simulink model "MATE_IEEE123Node"  (R2024b)
settings: Solver=FixedStepDiscrete  StartTime=0.0  StopTime=1  FixedStep=Ts  RelTol=1e-3
PostLoadFcn:
  | Ts=50e-6;init_IEEE123Node;
InitFcn:
  | Ts=50e-6;init_IEEE123Node;
undefined symbols (not defined in the file): ft2km, loadcoeff, MATE, MATERT, Pa1, Pa13, Pa14, Pa17, Pa18, Pa22, Pa24, Pa25, Pa29, Pa31, Pa32, Pa33, Pa34, Pa35, Pa37, Pa38, Pa39, Pa44, Pa46, Pa48, Pa50, Pa51, Pa52, Pa53, Pa57, Pa59, Pa6, Pa61, Pa67, Pa7, Pa70, Pa73, Pa8, Pa81, Pa82, Pa83, Pa84, Pa85, Pa9, Pb10, Pb15, Pb2, Pb30, Pb33, Pb34, Pb35, Pb41, Pb42, Pb43, Pb47, Pb48, Pb57, Pb58, Pb60, Pb65, Pb66 ... (+124)
libraries: simetranss x259, ee_lib x93, fl_lib x67, nesl_utility x67, simetran x2
(part 3 of 4)

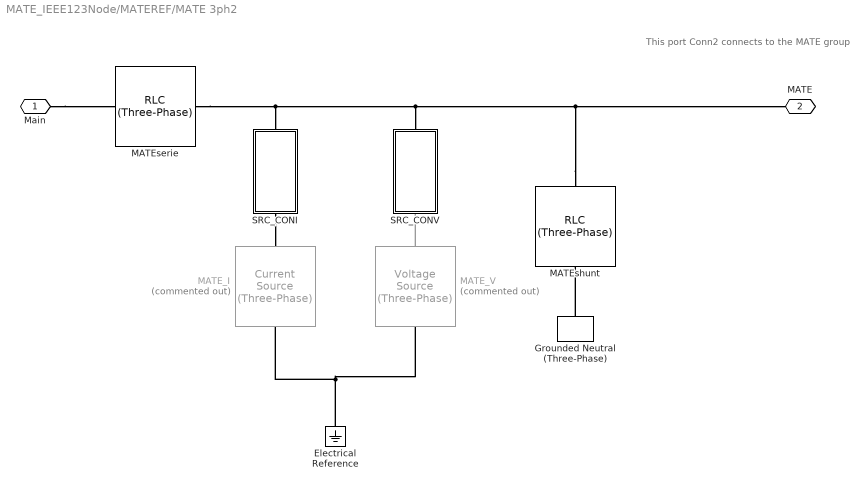
== system MATE_IEEE123Node/MATEREF/MATE 3ph2 ==
  note: This port Conn2 connects to the MATE group
  Electrical Reference : fl_lib/Electrical/Electrical Elements/Electrical Reference
  Grounded Neutral (Three-Phase) : ee_lib/Connectors & References/Grounded Neutral (Three-Phase)
  MATE_I : ee_lib/Sources/Current Source (Three-Phase)  Commented=on  iphase_rms=100 / sqrt(2) A  shift=0 deg  freq=60 Hz
      settings: InternalSimscapePortConfiguration="{\"Bottom\":[],\"Left\":[{\"id\":\"n\",\"label\":\"n\",\"type\":\"foundation.electrical.electrical\"}],\"Right\":[{\"id\":\"N\",\"label\":\"~\",\"type\":\"foundation.electrical.three_phase\"}],\"Top\":[]}"
  MATE_V : ee_lib/Sources/Voltage Source (Three-Phase)  Commented=on  vline_rms=0 V  shift=0 deg  freq=1 Hz  impedance_option=0  SShortCircuit=1e6 A*V  XR=15  R=0.0001 Ohm  L=3.97e-4 H  harmonic_option=0  harmonic_orders=[5, 7, 11, 13]  harmonic_ratios=[.1, .1, .1, .1]  G_parasitic=0 1/Ohm  I_specify=off  I_priority=None  I=[0, 0, 0] A  I_nominal_specify=off  I_nominal_value=1  I_nominal_unit=A
  MATEserie : ee_lib/Passive/RLC Assemblies/RLC (Three-Phase)  port_option=ee.enum.threePhasePort.composite  component_structure=ee.enum.rlc.structure.R  R=Rse Ohm  L=1e-3 H  C=1e-6 F  R_parasitic=0 Ohm  G_parasitic=0 1/Ohm  IL_specify=off  IL_priority=High  IL=[0, 0, 0] A  IL_nominal_specify=off  IL_nominal_value=1  IL_nominal_unit=A  VC_specify=off  VC_priority=High  VC=[0, 0, 0] V  VC_nominal_specify=off  VC_nominal_value=1  VC_nominal_unit=V
      settings: InternalSimscapePortConfiguration="{\"Bottom\":[],\"Left\":[{\"id\":\"N1\",\"label\":\"~1\",\"type\":\"foundation.electrical.three_phase\"}],\"Right\":[{\"id\":\"N2\",\"label\":\"~2\",\"type\":\"foundation.electrical.three_phase\"}],\"Top\":[]}"
  MATEshunt : ee_lib/Passive/RLC Assemblies/RLC (Three-Phase)  port_option=ee.enum.threePhasePort.composite  component_structure=ee.enum.rlc.structure.R  R=Rsh Ohm  L=1e-3 H  C=1e-6 F  R_parasitic=0 Ohm  G_parasitic=0 1/Ohm  IL_specify=off  IL_priority=High  IL=[0, 0, 0] A  IL_nominal_specify=off  IL_nominal_value=1  IL_nominal_unit=A  VC_specify=off  VC_priority=High  VC=[0, 0, 0] V  VC_nominal_specify=off  VC_nominal_value=1  VC_nominal_unit=V
      settings: InternalSimscapePortConfiguration="{\"Bottom\":[],\"Left\":[{\"id\":\"N1\",\"label\":\"~1\",\"type\":\"foundation.electrical.three_phase\"}],\"Right\":[{\"id\":\"N2\",\"label\":\"~2\",\"type\":\"foundation.electrical.three_phase\"}],\"Top\":[]}"
  SRC_CONI : Subsystem
  SRC_CONV : Subsystem
  Main : PMIOPort  Side=Left
  MATE : PMIOPort  Port=2  Side=Right
  connections:
  Main/RConn1 -- MATEserie/LConn1
  Grounded Neutral (Three-Phase)/LConn1 -- MATEshunt/LConn1
  SRC_CONI/RConn1 -- MATE_I/RConn1
  MATE_V/RConn1 -- SRC_CONV/RConn1
  MATE_V/LConn1 -- MATE_I/LConn1 -- Electrical Reference/LConn1
  MATEshunt/RConn1 -- MATE/RConn1 -- SRC_CONV/LConn1 -- MATEserie/RConn1 -- SRC_CONI/LConn1

== system MATE_IEEE123Node/MATEREF/sph ==
  Phase Splitter2 : ee_lib/Connectors & References/Phase Splitter
  abc : PMIOPort  Side=Left
  b : PMIOPort  Port=2  Side=Right
  connections:
  abc/RConn1 -- Phase Splitter2/LConn1
  b/RConn1 -- Phase Splitter2/RConn2

== system MATE_IEEE123Node/MATEREF/sph1 ==
  Phase Splitter2 : ee_lib/Connectors & References/Phase Splitter
  abc : PMIOPort  Side=Left
  b : PMIOPort  Port=2  Side=Right
  connections:
  b/RConn1 -- Phase Splitter2/RConn2
  abc/RConn1 -- Phase Splitter2/LConn1

== system MATE_IEEE123Node/MATEREF/sph2 ==
  Phase Splitter2 : ee_lib/Connectors & References/Phase Splitter
  abc : PMIOPort  Side=Left
  b : PMIOPort  Port=2  Side=Right
  connections:
  abc/RConn1 -- Phase Splitter2/LConn1
  b/RConn1 -- Phase Splitter2/RConn2

== system MATE_IEEE123Node/MATEREF/sph24 ==
  Phase Splitter2 : ee_lib/Connectors & References/Phase Splitter
  abc : PMIOPort  Side=Left
  c : PMIOPort  Port=2  Side=Right
  connections:
  abc/RConn1 -- Phase Splitter2/LConn1
  c/RConn1 -- Phase Splitter2/RConn3

== system MATE_IEEE123Node/MATEREF/sph25 ==
  Phase Splitter2 : ee_lib/Connectors & References/Phase Splitter
  abc : PMIOPort  Side=Left
  a : PMIOPort  Port=2  Side=Right
  connections:
  abc/RConn1 -- Phase Splitter2/LConn1
  a/RConn1 -- Phase Splitter2/RConn1

== system MATE_IEEE123Node/MATEREF/sph26 ==
  Phase Splitter2 : ee_lib/Connectors & References/Phase Splitter
  abc : PMIOPort  Side=Left
  b : PMIOPort  Port=2  Side=Right
  connections:
  abc/RConn1 -- Phase Splitter2/LConn1
  b/RConn1 -- Phase Splitter2/RConn2

== system MATE_IEEE123Node/MATEREF/sph27 ==
  Phase Splitter2 : ee_lib/Connectors & References/Phase Splitter
  abc : PMIOPort  Side=Left
  c : PMIOPort  Port=2  Side=Right
  connections:
  c/RConn1 -- Phase Splitter2/RConn3
  abc/RConn1 -- Phase Splitter2/LConn1

== system MATE_IEEE123Node/MATEREF/sph28 ==
  Phase Splitter2 : ee_lib/Connectors & References/Phase Splitter
  abc : PMIOPort  Side=Left
  b : PMIOPort  Port=2  Side=Right
  connections:
  b/RConn1 -- Phase Splitter2/RConn2
  abc/RConn1 -- Phase Splitter2/LConn1

== system MATE_IEEE123Node/MATEREF/sph29 ==
  Phase Splitter2 : ee_lib/Connectors & References/Phase Splitter
  abc : PMIOPort  Side=Left
  a : PMIOPort  Port=2  Side=Right
  connections:
  a/RConn1 -- Phase Splitter2/RConn1
  abc/RConn1 -- Phase Splitter2/LConn1

== system MATE_IEEE123Node/MATEREF/sph3 ==
  Phase Splitter2 : ee_lib/Connectors & References/Phase Splitter
  abc : PMIOPort  Side=Left
  b : PMIOPort  Port=2  Side=Right
  connections:
  abc/RConn1 -- Phase Splitter2/LConn1
  b/RConn1 -- Phase Splitter2/RConn2

== system MATE_IEEE123Node/MATEREF/sph30 ==
  Phase Splitter2 : ee_lib/Connectors & References/Phase Splitter
  abc : PMIOPort  Side=Left
  a : PMIOPort  Port=2  Side=Right
  connections:
  abc/RConn1 -- Phase Splitter2/LConn1
  a/RConn1 -- Phase Splitter2/RConn1

== system MATE_IEEE123Node/MATEREF/sph4 ==
  Phase Splitter2 : ee_lib/Connectors & References/Phase Splitter
  abc : PMIOPort  Side=Left
  b : PMIOPort  Port=2  Side=Right
  connections:
  b/RConn1 -- Phase Splitter2/RConn2
  abc/RConn1 -- Phase Splitter2/LConn1

== system MATE_IEEE123Node/MATEREF/sph42 ==
  Phase Splitter2 : ee_lib/Connectors & References/Phase Splitter
  abc : PMIOPort  Side=Left
  b : PMIOPort  Port=2  Side=Right
  connections:
  abc/RConn1 -- Phase Splitter2/LConn1
  b/RConn1 -- Phase Splitter2/RConn2

== system MATE_IEEE123Node/MATEREF/sph43 ==
  Phase Splitter2 : ee_lib/Connectors & References/Phase Splitter
  abc : PMIOPort  Side=Left
  a : PMIOPort  Port=2  Side=Right
  connections:
  a/RConn1 -- Phase Splitter2/RConn1
  abc/RConn1 -- Phase Splitter2/LConn1

== system MATE_IEEE123Node/MATEREF/sph44 ==
  Phase Splitter2 : ee_lib/Connectors & References/Phase Splitter
  abc : PMIOPort  Side=Left
  a : PMIOPort  Port=2  Side=Right
  connections:
  abc/RConn1 -- Phase Splitter2/LConn1
  a/RConn1 -- Phase Splitter2/RConn1

== system MATE_IEEE123Node/MATEREF/sph5 ==
  Phase Splitter2 : ee_lib/Connectors & References/Phase Splitter
  abc : PMIOPort  Side=Left
  c : PMIOPort  Port=2  Side=Right
  connections:
  abc/RConn1 -- Phase Splitter2/LConn1
  Phase Splitter2/RConn3 -- c/RConn1

== system MATE_IEEE123Node/MATEREF/sph51 ==
  Phase Splitter2 : ee_lib/Connectors & References/Phase Splitter
  abc : PMIOPort  Side=Left
  a : PMIOPort  Port=2  Side=Right
  connections:
  a/RConn1 -- Phase Splitter2/RConn1
  abc/RConn1 -- Phase Splitter2/LConn1

== system MATE_IEEE123Node/MATEREF/sph6 ==
  Phase Splitter2 : ee_lib/Connectors & References/Phase Splitter
  abc : PMIOPort  Side=Left
  a : PMIOPort  Port=2  Side=Right
  connections:
  abc/RConn1 -- Phase Splitter2/LConn1
  a/RConn1 -- Phase Splitter2/RConn1

== system MATE_IEEE123Node/MATEREF/sph7 ==
  Phase Splitter2 : ee_lib/Connectors & References/Phase Splitter
  abc : PMIOPort  Side=Left
  b : PMIOPort  Port=2  Side=Right
  connections:
  abc/RConn1 -- Phase Splitter2/LConn1
  b/RConn1 -- Phase Splitter2/RConn2

== system MATE_IEEE123Node/MATEREF/sph8 ==
  Phase Splitter2 : ee_lib/Connectors & References/Phase Splitter
  abc : PMIOPort  Side=Left
  a : PMIOPort  Port=2  Side=Right
  connections:
  a/RConn1 -- Phase Splitter2/RConn1
  abc/RConn1 -- Phase Splitter2/LConn1

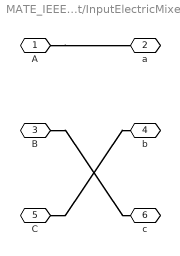
== system MATE_IEEE123Node/MATE_Equivalent/InputElectricMixer ==
  A : PMIOPort  Side=Left
  a : PMIOPort  Port=2  Side=Right
  B : PMIOPort  Port=3  Side=Left
  b : PMIOPort  Port=4  Side=Right
  C : PMIOPort  Port=5  Side=Left
  c : PMIOPort  Port=6  Side=Right
  connections:
  A/RConn1 -- a/RConn1
  B/RConn1 -- c/RConn1
  C/RConn1 -- b/RConn1

== system MATE_IEEE123Node/MATE_Equivalent/InternalSourceMixer ==
  0 : Constant  Value=-MATERT.SwitchVf./MATERT.Rsw  VectorParams1D=off
  1 : Constant  Value=ones(1,MATE.NumberOfNodes)  VectorParams1D=off
  Mux : Mux  Inputs=3
  Selector1 : Selector  Commented=on  InputPortWidth=size(MATE.source_parameter,1)+size(MATE.switch_parameter,1)  IndexOptions=Index vector (dialog)  Indices=MATE.src_Selector  OutputSizes=1
  sin : Sin  Amplitude=MATE.srcParam(1,:)  Frequency=MATE.srcParam(3,:)*2*pi  Phase=MATE.srcParam(2,:)*pi/180  SampleTime=Ts
  Out1 : Outport
  wires:
  sin/1 -> Mux/2
  0/1 -> Mux/1
  Mux/1 -> Out1/1
  1/1 -> Mux/3

== system MATE_IEEE123Node/MATE_Equivalent/InternalSwitchMixer ==
  Mux2 : Mux  Inputs=2
  Selector7 : Selector  InputPortWidth=1  IndexOptions=Index vector (dialog)  Indices="[ 1  1  1 ]"  OutputSizes=1
  gate : Outport
  wires:
  Selector7/1 -> Mux2/1
  [a58fxa8a9x743c756a9e3e] -> Selector7/1
  Mux2/1 -> gate/1
  [ae38xba66x2f62aef96d10] -> Mux2/2

== system MATE_IEEE123Node/MATE_Equivalent/MATEOutputSelector ==
  Yout : Inport
  BusCreator : BusCreator  Inputs=25
  Demux : Demux  Outputs=25
  SigOut : Outport
  wires:
  Demux/1 -> BusCreator/1  "SW_voltage:_1_CircuitBreaker3ph"
  Demux/2 -> BusCreator/2  "SW_voltage:_2_CircuitBreaker3ph"
  Demux/3 -> BusCreator/3  "SW_voltage:_3_CircuitBreaker3ph"
  Demux/4 -> BusCreator/4  "SW_voltage:_4_Switch"
  Demux/5 -> BusCreator/5  "Voltage:_5_CV_xfo"
  Demux/6 -> BusCreator/6  "Voltage:_6_CV_xfo"
  Demux/7 -> BusCreator/7  "Voltage:_7_CV_xfo"
  Demux/8 -> BusCreator/8  "Voltage:_8_bus13VI"
  Demux/9 -> BusCreator/9  "Voltage:_9_bus13VI"
  Demux/10 -> BusCreator/10  "Voltage:_10_bus13VI"
  Demux/11 -> BusCreator/11  "current:_11_CV_xfo"
  Demux/12 -> BusCreator/12  "current:_12_CV_xfo"
  Demux/13 -> BusCreator/13  "current:_13_CV_xfo"
  Demux/14 -> BusCreator/14  "current:_14_bus13VI"
  Demux/15 -> BusCreator/15  "current:_15_bus13VI"
  Demux/16 -> BusCreator/16  "current:_16_bus13VI"
  Demux/17 -> BusCreator/17  "MATEOut:_17_internal"
  Demux/18 -> BusCreator/18  "MATEOut:_18_internal"
  Demux/19 -> BusCreator/19  "MATEOut:_19_internal"
  Demux/20 -> BusCreator/20  "MATEOut:_20_internal"
  Demux/21 -> BusCreator/21  "MATEOut:_21_internal"
  Demux/22 -> BusCreator/22  "MATEOut:_22_internal"
  Demux/23 -> BusCreator/23  "MATEOut:_23_internal"
  Demux/24 -> BusCreator/24  "MATEOut:_24_internal"
  Demux/25 -> BusCreator/25  "MATEOut:_25_internal"
  BusCreator/1 -> SigOut/1
  Yout/1 -> Demux/1

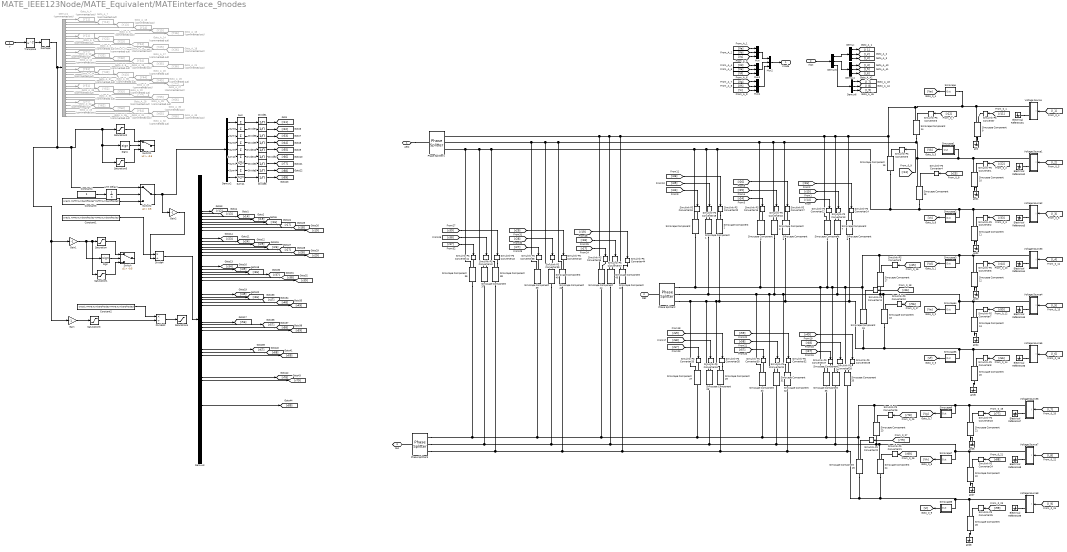
== system MATE_IEEE123Node/MATE_Equivalent/MATEinterface_9nodes ==
  Y : Inport
  Ihist : Inport  Port=2
  Constant1 : Constant  Value=ones(1,MATE.NumberOfNodes*MATE.NumberOfNodes)
  Constant2 : Constant  Value=ones(1,MATE.NumberOfNodes*MATE.NumberOfNodes)
  Constant3 : Constant  Value=ones(1,MATE.NumberOfNodes*MATE.NumberOfNodes)
  Constant4 : Constant
  Demux : Demux  Outputs=3
      settings: DisplayOption=none
  Demux1 : Demux  Commented=on  Outputs=36
      settings: DisplayOption=none
  Demux2 : Demux  Outputs="[9 9 9  9 9 9  9 9 9]"
      settings: DisplayOption=none
  Demux3 : Demux  Outputs=81
      settings: DisplayOption=none
  Demux4 : Demux  Outputs=3
      settings: DisplayOption=none
  Demux5 : Demux  Outputs=[3 3 3]
      settings: DisplayOption=none
  Demux6 : Demux  Outputs=3
      settings: DisplayOption=none
  Divide{1..3,5..11} (10 alike) : Product  Inputs=/
  Divide12 : Product  Inputs=*/  CollapseMode=Specified dimension
  Divide4 : Product  Inputs=*/  CollapseMode=Specified dimension
  Electrical Reference{1..9} (9 alike) : fl_lib/Electrical/Electrical Elements/Electrical Reference
  Gain : Gain  Gain=-1
  Gain1 : Gain  Gain=-1
  Gain2 : Gain  Gain=-1
  Goto_A_10 : Goto  Commented=on  GotoTag=Y23
  Goto_A_11 : Goto  Commented=on  GotoTag=Y31
  Goto_A_12 : Goto  Commented=on  GotoTag=Y32
  Goto_A_13 : Goto  Commented=on  GotoTag=Y14
  Goto_A_14 : Goto  Commented=on  GotoTag=Y15
  Goto_A_15 : Goto  Commented=on  GotoTag=Y16
  Goto_A_16 : Goto  Commented=on  GotoTag=Y24
  Goto_A_17 : Goto  Commented=on  GotoTag=Y25
  Goto_A_18 : Goto  Commented=on  GotoTag=Y26
  Goto_A_19 : Goto  Commented=on  GotoTag=Y34
  Goto_A_20 : Goto  Commented=on  GotoTag=Y35
  Goto_A_21 : Goto  Commented=on  GotoTag=Y36
  Goto_A_22 : Goto  Commented=on  GotoTag=Y53
  Goto_A_23 : Goto  Commented=on  GotoTag=Y61
  Goto_A_24 : Goto  Commented=on  GotoTag=Y62
  Goto_A_25 : Goto  Commented=on  GotoTag=Y44
  Goto_A_26 : Goto  Commented=on  GotoTag=Y45
  Goto_A_27 : Goto  Commented=on  GotoTag=Y46
  Goto_A_28 : Goto  Commented=on  GotoTag=Y54
  Goto_A_29 : Goto  Commented=on  GotoTag=Y55
  Goto_A_30 : Goto  Commented=on  GotoTag=Y66
  Goto_A_31 : Goto  Commented=on  GotoTag=Y64
  Goto_A_32 : Goto  Commented=on  GotoTag=Y65
  Goto_A_33 : Goto  Commented=on  GotoTag=Y66
  Goto_A_34 : Goto  Commented=on  GotoTag=Y41
  Goto_A_35 : Goto  Commented=on  GotoTag=Y52
  Goto_A_36 : Goto  Commented=on  GotoTag=Y63
  Goto_A_37 : Goto  Commented=on  GotoTag=Y42
  Goto_A_38 : Goto  Commented=on  GotoTag=Y43
  Goto_A_39 : Goto  Commented=on  GotoTag=Y51
  Goto_A_4 : Goto  Commented=on  GotoTag=Y11
  Goto_A_5 : Goto  Commented=on  GotoTag=Y22
  Goto_A_6 : Goto  Commented=on  GotoTag=Y33
  Goto_A_7 : Goto  Commented=on  GotoTag=Y12
  Goto_A_8 : Goto  Commented=on  GotoTag=Y13
  Goto_A_9 : Goto  Commented=on  GotoTag=Y21
  Mux : Mux  Inputs=3
  Mux1 : Mux  Inputs=3
  Mux2 : Mux  Inputs=[3 3 3]
  Mux4 : Mux  Inputs=3
  Phase Splitter1 : ee_lib/Connectors & References/Phase Splitter
  Phase Splitter2 : ee_lib/Connectors & References/Phase Splitter
  Phase Splitter3 : ee_lib/Connectors & References/Phase Splitter
  Reshape : Reshape
  Saturation : Saturate  UpperLimit=1e12  LowerLimit=1e-12
  Saturation1 : Saturate  UpperLimit=-1e-12  LowerLimit=-1e12
  Saturation2 : Saturate  UpperLimit=1e12  LowerLimit=1e-12
  Saturation3 : Saturate  UpperLimit=1e15  LowerLimit=-1e15
  Saturation4 : Saturate  UpperLimit=1e15  LowerLimit=-1e15
  Saturation5 : Saturate  UpperLimit=-1e-12  LowerLimit=-1e12
  Sign : Signum
  Sign1 : Signum
  Simscape : Subsystem
      mask Display: disp('V')
  Simscape Component{,1..44} (45 alike) : SimscapeComponentBlock  SourceFile=variable_resistor_unlimited  ComponentPath=variable_resistor_unlimited  ComponentVariants="[\"variable_resistor_unlimited\"]"  ComponentVariantNames="[\"variable_resistor_unlimited\"]"  ClassName=variable_resistor_unlimited  SchemaVersion=1  R0=0 Ohm  Rmaxp=1e9 Ohm  Rmaxn=-1e9 Ohm  Rminp=1e-9 Ohm  Rminn=-1e-9 Ohm  i_specify=off  i_priority=None  i=0 A  i_nominal_specify=off  i_nominal_value=1  i_nominal_unit=A  v_specify=off  v_priority=None  v=0 V  v_nominal_specify=off  v_nominal_value=1  v_nominal_unit=V
      settings: CopyFcn=simscape.engine.sli.internal.componentblockcallback(gcbh,'COPY')  PreCopyFcn=simscape.engine.sli.internal.componentblockcallback(gcbh,'PRECOPY')  PreDeleteFcn=simscape.engine.sli.internal.componentblockcallback(gcbh,'PREDELETE')  InternalSimscapePortConfiguration="{\"Bottom\":[],\"Left\":[{\"id\":\"R\",\"label\":\"R\",\"type\":\"input\"},{\"id\":\"p\",\"label\":\"+\",\"type\":\"foundation.electrical.electrical\"}],\"Right\":[{\"id\":\"n\",\"label\":\"-\",\"type\":\"foundation.electrical.electrical\"}],\"Top\":[]}"
      mask Type: Variable Resistor
  Simscape1 : Subsystem
      mask Display: disp('V')
  Simscape2 : Subsystem
      mask Display: disp('V')
  Simscape3 : Subsystem
      mask Display: disp('V')
  Simscape4 : Subsystem
      mask Display: disp('V')
  Simscape5 : Subsystem
      mask Display: disp('V')
  Simscape6 : Subsystem
      mask Display: disp('V')
  Simscape7 : Subsystem
      mask Display: disp('V')
  Simscape8 : Subsystem
      mask Display: disp('V')
  Simulink-PS Converter{,1..44} (45 alike) : nesl_utility/Simulink-PS Converter  PhysicalDomain=network_engine_domain  SubClassName=ps_input  LeftPortType=input  RightPortType=output  PseudoPeriodic=off  Frequencies=[]  NoiseDistribution=none  NoiseParameters=[]  Unit=1  AffineConversion=off  FilteringAndDerivatives=provide  SimscapeFilterOrder=1  InputFilterTimeConstant=0.001  UdotUserProvided=0
  Sum{,1..2,4..11} (11 alike) : Sum  Inputs=+
  Switch : Switch  Criteria=u2 > Threshold  Threshold=-0.5  SaturateOnIntegerOverflow=off  InputSameDT=off
  Switch1 : Switch  Criteria=u2 > Threshold  Threshold=-0.5  SaturateOnIntegerOverflow=off  InputSameDT=off
  Switch2 : Switch  Criteria=u2 > Threshold  Threshold=0.5  SaturateOnIntegerOverflow=off  InputSameDT=off
  Transpose : Math  Operator=transpose
  Unit Delay1 : UnitDelay  SampleTime=Ts  HasFrameUpgradeWarning=on
  Voltage Source : Subsystem
  Voltage Source1 : Subsystem
  Voltage Source2 : Subsystem
  Voltage Source3 : Subsystem
  Voltage Source4 : Subsystem
  Voltage Source5 : Subsystem
  Voltage Source6 : Subsystem
  Voltage Source7 : Subsystem
  Voltage Source8 : Subsystem
  gnd{,1..8} (9 alike) : fl_lib/Electrical/Electrical Elements/Electrical Reference
  ABC : PMIOPort  Side=Right
  DEF : PMIOPort  Port=2  Side=Right
  GHI : PMIOPort  Port=3  Side=Right
  Vnode : Outport  VectorParamsAs1DForOutWhenUnconnected=off
  wires:
  Demux/3 -> [I_3]
  [Vc] -> Mux/3
  Demux/2 -> [I_2]
  [Vb] -> Mux/2
  Demux/1 -> [I_1]
  [Va] -> Mux/1
  [I_2] -> Voltage Source1/1(I)
  Simscape2/1(Out) -> [Vc]
  [I_3] -> Voltage Source2/1(I)
  Simscape/1(Out) -> [Va]
  Simscape1/1(Out) -> [Vb]
  [I_1] -> Voltage Source/1(I)
  Y/1 -> Transpose/1
  Demux1/1 -> Goto_A_4/1
  Demux1/2 -> Goto_A_7/1
  Demux1/3 -> Goto_A_8/1
  Transpose/1 -> Reshape/1
  [r11] -> Simulink-PS Converter/1
  Sum/1 -> Divide1/1
  Divide1/1 -> [r11]
  [r22] -> Simulink-PS Converter1/1
  [r33] -> Simulink-PS Converter2/1
  [r12] -> Simulink-PS Converter3/1
  [r23] -> Simulink-PS Converter4/1
  [r13] -> Simulink-PS Converter5/1
  Demux1/4 -> Goto_A_13/1
  Demux1/5 -> Goto_A_14/1
  Demux1/6 -> Goto_A_15/1
  Demux1/7 -> Goto_A_9/1
  Demux1/8 -> Goto_A_5/1
  Demux1/9 -> Goto_A_10/1
  Demux1/10 -> Goto_A_16/1
  Demux1/11 -> Goto_A_17/1
  Demux1/12 -> Goto_A_18/1
  Demux1/13 -> Goto_A_11/1
  Demux1/14 -> Goto_A_12/1
  Demux1/15 -> Goto_A_6/1
  Demux1/16 -> Goto_A_19/1
  Demux1/17 -> Goto_A_20/1
  Demux1/18 -> Goto_A_21/1
  Demux1/36 -> Goto_A_33/1
  Demux1/35 -> Goto_A_32/1
  Demux1/34 -> Goto_A_31/1
  Demux1/33 -> Goto_A_36/1
  Demux1/32 -> Goto_A_24/1
  Demux1/31 -> Goto_A_23/1
  Demux1/30 -> Goto_A_30/1
  Demux1/29 -> Goto_A_29/1
  Demux1/28 -> Goto_A_28/1
  Demux1/27 -> Goto_A_22/1
  Demux1/26 -> Goto_A_35/1
  Demux1/25 -> Goto_A_39/1
  Demux1/24 -> Goto_A_27/1
  Demux1/23 -> Goto_A_26/1
  Demux1/22 -> Goto_A_25/1
  Demux1/21 -> Goto_A_38/1
  Demux1/20 -> Goto_A_37/1
  Demux1/19 -> Goto_A_34/1
  Demux2/1 -> Sum/1
  Divide7/1 -> [r22]
  Sum6/1 -> Divide7/1
  Demux2/2 -> Sum6/1
  Sum7/1 -> Divide8/1
  Divide8/1 -> [r33]
  Demux2/3 -> Sum7/1
  Demux2/4 -> Sum8/1
  Divide9/1 -> [r44]
  Sum8/1 -> Divide9/1
  Sum9/1 -> Divide10/1
  Divide10/1 -> [r55]
  Demux2/5 -> Sum9/1
  Divide11/1 -> [r66]
  Sum10/1 -> Divide11/1
  Demux2/6 -> Sum10/1
  [r44] -> Simulink-PS Converter6/1
  [I_4] -> Voltage Source3/1(I)
  Simscape3/1(Out) -> [Vd]
  Simscape4/1(Out) -> [Ve]
  [I_5] -> Voltage Source4/1(I)
  [r55] -> Simulink-PS Converter7/1
  [r66] -> Simulink-PS Converter8/1
  [I_6] -> Voltage Source5/1(I)
  Simscape5/1(Out) -> [Vf]
  [r45] -> Simulink-PS Converter9/1
  [r56] -> Simulink-PS Converter10/1
  [r46] -> Simulink-PS Converter11/1
  [Vd] -> Mux1/1
  [Ve] -> Mux1/2
  [Vf] -> Mux1/3
  Demux4/1 -> [I_4]
  Demux4/2 -> [I_5]
  Demux4/3 -> [I_6]
  [r14] -> Simulink-PS Converter12/1
  [r15] -> Simulink-PS Converter13/1
  [r16] -> Simulink-PS Converter14/1
  [r26] -> Simulink-PS Converter17/1
  [r25] -> Simulink-PS Converter16/1
  [r24] -> Simulink-PS Converter15/1
  Mux/1 -> Mux2/1
  Mux1/1 -> Mux2/2
  Mux2/1 -> Vnode/1
  Ihist/1 -> Demux5/1
  Demux5/1 -> Demux/1
  Demux5/2 -> Demux4/1
  Demux3/2 -> [r12]
  Demux3/3 -> [r13]
  Demux3/4 -> [r14]
  Demux3/5 -> [r15]
  Demux3/6 -> [r16]
  Gain1/1 -> Sign/1, Saturation1/1, Saturation/1
  Constant1/1 -> Divide4/1
  [r36] -> Simulink-PS Converter20/1
  [r35] -> Simulink-PS Converter19/1
  [r34] -> Simulink-PS Converter18/1
  Sign/1 -> Switch/2
  Saturation/1 -> Switch/1
  Saturation1/1 -> Switch/3
  Sum1/1 -> Divide3/1
  Divide3/1 -> [r77]
  Demux2/7 -> Sum1/1
  Divide5/1 -> [r88]
  Sum4/1 -> Divide5/1
  Demux2/8 -> Sum4/1
  Sum11/1 -> Divide6/1
  Divide6/1 -> [r99]
  Demux2/9 -> Sum11/1
  Demux3/7 -> [r17]
  Demux3/8 -> [r18]
  Demux3/9 -> [r19]
  Demux3/12 -> [r23]
  Demux3/13 -> [r24]
  Demux3/14 -> [r25]
  Demux3/15 -> [r26]
  Demux3/18 -> [r29]
  Demux3/17 -> [r28]
  Demux3/16 -> [r27]
  Demux3/22 -> [r34]
  Demux3/23 -> [r35]
  Demux3/24 -> [r36]
  Demux3/25 -> [r37]
  Demux3/26 -> [r38]
  Demux3/27 -> [r39]
  Demux3/32 -> [r45]
  Demux3/33 -> [r46]
  Demux3/36 -> [r49]
  Demux3/35 -> [r48]
  Demux3/34 -> [r47]
  Demux3/42 -> [r56]
  Demux3/44 -> [r58]
  Demux3/45 -> [r59]
  Demux3/43 -> [r57]
  Demux3/54 -> [r69]
  Demux3/53 -> [r68]
  Demux3/52 -> [r67]
  Demux3/63 -> [r79]
  Demux3/62 -> [r78]
  Demux3/72 -> [r89]
  Mux4/1 -> Mux2/3
  [Vi] -> Mux4/3
  [Vh] -> Mux4/2
  [Vg] -> Mux4/1
  Demux6/3 -> [I_9]
  Demux6/2 -> [I_8]
  Demux6/1 -> [I_7]
  Demux5/3 -> Demux6/1
  [r79] -> Simulink-PS Converter22/1
  [r89] -> Simulink-PS Converter21/1
  [r78] -> Simulink-PS Converter26/1
  Simscape8/1(Out) -> [Vi]
  [I_9] -> Voltage Source8/1(I)
  [r99] -> Simulink-PS Converter25/1
  [r88] -> Simulink-PS Converter24/1
  [I_8] -> Voltage Source7/1(I)
  Simscape7/1(Out) -> [Vh]
  Simscape6/1(Out) -> [Vg]
  [I_7] -> Voltage Source6/1(I)
  [r77] -> Simulink-PS Converter23/1
  [r67] -> Simulink-PS Converter33/1
  [r68] -> Simulink-PS Converter34/1
  [r69] -> Simulink-PS Converter35/1
  [r57] -> Simulink-PS Converter30/1
  [r58] -> Simulink-PS Converter31/1
  [r59] -> Simulink-PS Converter32/1
  [r49] -> Simulink-PS Converter29/1
  [r48] -> Simulink-PS Converter28/1
  [r47] -> Simulink-PS Converter27/1
  [r17] -> Simulink-PS Converter36/1
  [r18] -> Simulink-PS Converter37/1
  [r19] -> Simulink-PS Converter44/1
  [r29] -> Simulink-PS Converter40/1
  [r28] -> Simulink-PS Converter39/1
  [r27] -> Simulink-PS Converter38/1
  [r39] -> Simulink-PS Converter43/1
  [r38] -> Simulink-PS Converter42/1
  [r37] -> Simulink-PS Converter41/1
  Divide12/1 -> Saturation4/1
  Saturation3/1 -> Divide12/2
  Constant2/1 -> Divide12/1
  Gain/1 -> Saturation3/1
  Divide4/1 -> Demux3/1
  Saturation5/1 -> Switch1/3
  Saturation2/1 -> Switch1/1
  Sign1/1 -> Switch1/2
  Reshape/1 -> Gain1/1, Gain/1, Saturation5/1, Sign1/1, Saturation2/1, Switch2/1, Demux1/1
  Switch2/1 -> Gain2/1, Demux2/1
  Unit Delay1/1 -> Switch2/2
  Constant4/1 -> Unit Delay1/1
  Constant3/1 -> Switch2/3
  Gain2/1 -> Divide4/2
  connections:
  Simscape Component14/LConn2 -- Simscape Component9/LConn2 -- Voltage Source/RConn1 -- Simscape/LConn1 -- Simscape Component16/LConn2 -- Simscape Component6/LConn2 -- Simscape Component7/LConn2 -- Simscape Component8/LConn2 -- Simscape Component42/LConn2 -- Simscape Component43/LConn2 -- Simscape Component44/LConn2 -- Phase Splitter1/RConn1
  Simscape Component11/LConn2 -- Voltage Source2/RConn1 -- Simscape2/LConn1 -- Simscape Component15/RConn1 -- Simscape Component16/RConn1 -- Simscape Component2/LConn2 -- Simscape Component1/LConn2 -- Simscape Component/LConn2 -- Simscape Component38/LConn2 -- Simscape Component37/LConn2 -- Simscape Component36/LConn2 -- Phase Splitter1/RConn3
  Simscape Component10/LConn2 -- Voltage Source1/RConn1 -- Simscape1/LConn1 -- Simscape Component15/LConn2 -- Simscape Component14/RConn1 -- Simscape Component5/LConn2 -- Simscape Component4/LConn2 -- Simscape Component3/LConn2 -- Simscape Component41/LConn2 -- Simscape Component40/LConn2 -- Simscape Component39/LConn2 -- Phase Splitter1/RConn2
  Electrical Reference2/LConn1 -- Voltage Source1/RConn2
  Electrical Reference3/LConn1 -- Voltage Source2/RConn2
  Electrical Reference1/LConn1 -- Voltage Source/RConn2
  ABC/RConn1 -- Phase Splitter1/LConn1
  Simscape Component9/RConn1 -- gnd/LConn1
  Simscape Component9/LConn1 -- Simulink-PS Converter/RConn1
  Simscape Component10/RConn1 -- gnd1/LConn1
  Simscape Component10/LConn1 -- Simulink-PS Converter1/RConn1
  Simscape Component11/RConn1 -- gnd2/LConn1
  Simscape Component11/LConn1 -- Simulink-PS Converter2/RConn1
  Simscape Component14/LConn1 -- Simulink-PS Converter3/RConn1
  Simscape Component15/LConn1 -- Simulink-PS Converter4/RConn1
  Simscape Component16/LConn1 -- Simulink-PS Converter5/RConn1
  Simscape Component17/LConn2 -- Simscape Component3/RConn1 -- Simscape Component/RConn1 -- Phase Splitter2/RConn1 -- Simscape Component35/LConn2 -- Simscape Component8/RConn1 -- Simscape Component34/LConn2 -- Simscape Component33/LConn2 -- Simscape Component19/LConn2 -- Simscape Component12/LConn2 -- Voltage Source3/RConn1 -- Simscape3/LConn1
  Simscape Component12/LConn1 -- Simulink-PS Converter6/RConn1
  Simscape Component12/RConn1 -- gnd3/LConn1
  Electrical Reference4/LConn1 -- Voltage Source3/RConn2
  Simscape Component13/LConn2 -- Voltage Source4/RConn1 -- Simscape4/LConn1 -- Simscape Component17/RConn1 -- Simscape Component1/RConn1 -- Phase Splitter2/RConn2 -- Simscape Component30/LConn2 -- Simscape Component31/LConn2 -- Simscape Component4/RConn1 -- Simscape Component32/LConn2 -- Simscape Component7/RConn1 -- Simscape Component18/LConn2
  Simscape Component13/RConn1 -- gnd4/LConn1
  Simscape Component13/LConn1 -- Simulink-PS Converter7/RConn1
  Electrical Reference5/LConn1 -- Voltage Source4/RConn2
  Simscape Component6/RConn1 -- Phase Splitter2/RConn3 -- Simscape Component27/LConn2 -- Simscape Component28/LConn2 -- Simscape Component29/LConn2 -- Simscape Component2/RConn1 -- Simscape Component5/RConn1 -- Simscape Component19/RConn1 -- Simscape Component18/RConn1 -- Simscape5/LConn1 -- Voltage Source5/RConn1 -- Simscape Component20/LConn2
  Electrical Reference6/LConn1 -- Voltage Source5/RConn2
  Simscape Component20/LConn1 -- Simulink-PS Converter8/RConn1
  Simscape Component20/RConn1 -- gnd5/LConn1
  Phase Splitter2/LConn1 -- DEF/RConn1
  Simscape Component17/LConn1 -- Simulink-PS Converter9/RConn1
  Simscape Component18/LConn1 -- Simulink-PS Converter10/RConn1
  Simscape Component19/LConn1 -- Simulink-PS Converter11/RConn1
  Simscape Component8/LConn1 -- Simulink-PS Converter12/RConn1
  Simscape Component7/LConn1 -- Simulink-PS Converter13/RConn1
  Simscape Component6/LConn1 -- Simulink-PS Converter14/RConn1
  Simscape Component3/LConn1 -- Simulink-PS Converter15/RConn1
  Simscape Component4/LConn1 -- Simulink-PS Converter16/RConn1
  Simscape Component5/LConn1 -- Simulink-PS Converter17/RConn1
  Simscape Component/LConn1 -- Simulink-PS Converter18/RConn1
  Simscape Component1/LConn1 -- Simulink-PS Converter19/RConn1
  Simulink-PS Converter20/RConn1 -- Simscape Component2/LConn1
  Simscape Component23/LConn2 -- Simscape Component36/RConn1 -- Phase Splitter3/RConn1 -- Simscape Component39/RConn1 -- Simscape Component44/RConn1 -- Simscape Component27/RConn1 -- Simscape Component30/RConn1 -- Simscape Component35/RConn1 -- Simscape Component25/LConn2 -- Simscape6/LConn1 -- Voltage Source6/RConn1 -- Simscape Component21/LConn2
  Simscape Component22/LConn2 -- Simscape Component24/LConn2 -- Simscape Component37/RConn1 -- Phase Splitter3/RConn2 -- Simscape Component40/RConn1 -- Simscape Component43/RConn1 -- Simscape Component28/RConn1 -- Simscape Component31/RConn1 -- Simscape Component34/RConn1 -- Simscape Component23/RConn1 -- Simscape7/LConn1 -- Voltage Source7/RConn1
  Simscape Component25/RConn1 -- Phase Splitter3/RConn3 -- Simscape Component38/RConn1 -- Simscape Component41/RConn1 -- Simscape Component42/RConn1 -- Simscape Component29/RConn1 -- Simscape Component32/RConn1 -- Simscape Component33/RConn1 -- Simscape Component26/LConn2 -- Voltage Source8/RConn1 -- Simscape8/LConn1 -- Simscape Component24/RConn1
  Simscape Component25/LConn1 -- Simulink-PS Converter22/RConn1
  Simscape Component23/LConn1 -- Simulink-PS Converter26/RConn1
  Simscape Component26/RConn1 -- gnd8/LConn1
  Electrical Reference9/LConn1 -- Voltage Source8/RConn2
  Simscape Component22/RConn1 -- gnd7/LConn1
  Electrical Reference7/LConn1 -- Voltage Source6/RConn2
  Electrical Reference8/LConn1 -- Voltage Source7/RConn2
  Simscape Component21/RConn1 -- gnd6/LConn1
  Simscape Component26/LConn1 -- Simulink-PS Converter25/RConn1
  Simscape Component24/LConn1 -- Simulink-PS Converter21/RConn1
  Simscape Component21/LConn1 -- Simulink-PS Converter23/RConn1
  Simscape Component22/LConn1 -- Simulink-PS Converter24/RConn1
  Phase Splitter3/LConn1 -- GHI/RConn1
  Simscape Component28/LConn1 -- Simulink-PS Converter34/RConn1
  Simscape Component27/LConn1 -- Simulink-PS Converter33/RConn1
  Simscape Component32/LConn1 -- Simulink-PS Converter32/RConn1
  Simscape Component31/LConn1 -- Simulink-PS Converter31/RConn1
  Simscape Component30/LConn1 -- Simulink-PS Converter30/RConn1
  Simscape Component33/LConn1 -- Simulink-PS Converter29/RConn1
  Simscape Component34/LConn1 -- Simulink-PS Converter28/RConn1
  Simscape Component35/LConn1 -- Simulink-PS Converter27/RConn1
  Simulink-PS Converter35/RConn1 -- Simscape Component29/LConn1
  Simulink-PS Converter43/RConn1 -- Simscape Component38/LConn1
  Simscape Component44/LConn1 -- Simulink-PS Converter36/RConn1
  Simulink-PS Converter44/RConn1 -- Simscape Component42/LConn1
  Simscape Component39/LConn1 -- Simulink-PS Converter38/RConn1
  Simscape Component40/LConn1 -- Simulink-PS Converter39/RConn1
  Simscape Component41/LConn1 -- Simulink-PS Converter40/RConn1
  Simscape Component36/LConn1 -- Simulink-PS Converter41/RConn1
  Simscape Component43/LConn1 -- Simulink-PS Converter37/RConn1
  Simscape Component37/LConn1 -- Simulink-PS Converter42/RConn1

== system MATE_IEEE123Node/NorthEast/28 ==
  Connection Port : PMIOPort  Side=Left
  Connection Port1 : PMIOPort  Port=2  Side=Right
  Connection Port2 : PMIOPort  Port=3  Side=Left
  Connection Port3 : PMIOPort  Port=4  Side=Right
  connections:
  Connection Port/RConn1 -- Connection Port1/RConn1
  Connection Port2/RConn1 -- Connection Port3/RConn1

== system MATE_IEEE123Node/NorthEast/sph21 ==
  Phase Splitter2 : ee_lib/Connectors & References/Phase Splitter
  abc : PMIOPort  Side=Left
  a : PMIOPort  Port=2  Side=Right
  connections:
  Phase Splitter2/RConn1 -- a/RConn1
  abc/RConn1 -- Phase Splitter2/LConn1

== system MATE_IEEE123Node/NorthEast/sph22 ==
  Phase Splitter2 : ee_lib/Connectors & References/Phase Splitter
  abc : PMIOPort  Side=Left
  a : PMIOPort  Port=2  Side=Right
  connections:
  abc/RConn1 -- Phase Splitter2/LConn1
  a/RConn1 -- Phase Splitter2/RConn1

== system MATE_IEEE123Node/NorthEast/sph23 ==
  Phase Splitter2 : ee_lib/Connectors & References/Phase Splitter
  abc : PMIOPort  Side=Left
  c : PMIOPort  Port=2  Side=Right
  connections:
  abc/RConn1 -- Phase Splitter2/LConn1
  Phase Splitter2/RConn3 -- c/RConn1

== system MATE_IEEE123Node/NorthEast/sph31 ==
  Phase Splitter2 : ee_lib/Connectors & References/Phase Splitter
  abc : PMIOPort  Side=Left
  a : PMIOPort  Port=2  Side=Right
  connections:
  abc/RConn1 -- Phase Splitter2/LConn1
  a/RConn1 -- Phase Splitter2/RConn1

== system MATE_IEEE123Node/NorthEast/sph32 ==
  Phase Splitter2 : ee_lib/Connectors & References/Phase Splitter
  abc : PMIOPort  Side=Left
  b : PMIOPort  Port=2  Side=Right
  connections:
  abc/RConn1 -- Phase Splitter2/LConn1
  Phase Splitter2/RConn2 -- b/RConn1

== system MATE_IEEE123Node/NorthEast/sph33 ==
  Phase Splitter2 : ee_lib/Connectors & References/Phase Splitter
  abc : PMIOPort  Side=Left
  c : PMIOPort  Port=2  Side=Right
  connections:
  abc/RConn1 -- Phase Splitter2/LConn1
  Phase Splitter2/RConn3 -- c/RConn1

== system MATE_IEEE123Node/NorthEast/sph34 ==
  Phase Splitter2 : ee_lib/Connectors & References/Phase Splitter
  abc : PMIOPort  Side=Left
  a : PMIOPort  Port=2  Side=Right
  c : PMIOPort  Port=3  Side=Right
  connections:
  Phase Splitter2/RConn3 -- c/RConn1
  abc/RConn1 -- Phase Splitter2/LConn1
  a/RConn1 -- Phase Splitter2/RConn1

== system MATE_IEEE123Node/NorthEast/sph35 ==
  Phase Splitter2 : ee_lib/Connectors & References/Phase Splitter
  abc : PMIOPort  Side=Left
  a : PMIOPort  Port=2  Side=Right
  connections:
  a/RConn1 -- Phase Splitter2/RConn1
  abc/RConn1 -- Phase Splitter2/LConn1

== system MATE_IEEE123Node/NorthEast/sph36 ==
  Phase Splitter2 : ee_lib/Connectors & References/Phase Splitter
  abc : PMIOPort  Side=Left
  a : PMIOPort  Port=2  Side=Right
  connections:
  abc/RConn1 -- Phase Splitter2/LConn1
  a/RConn1 -- Phase Splitter2/RConn1

== system MATE_IEEE123Node/NorthEast/sph37 ==
  Phase Splitter2 : ee_lib/Connectors & References/Phase Splitter
  abc : PMIOPort  Side=Left
  c : PMIOPort  Port=2  Side=Right
  connections:
  abc/RConn1 -- Phase Splitter2/LConn1
  Phase Splitter2/RConn3 -- c/RConn1

== system MATE_IEEE123Node/NorthEast/sph38 ==
  Phase Splitter2 : ee_lib/Connectors & References/Phase Splitter
  abc : PMIOPort  Side=Left
  c : PMIOPort  Port=2  Side=Right
  connections:
  abc/RConn1 -- Phase Splitter2/LConn1
  c/RConn1 -- Phase Splitter2/RConn3

== system MATE_IEEE123Node/NorthEast/sph39 ==
  Phase Splitter2 : ee_lib/Connectors & References/Phase Splitter
  abc : PMIOPort  Side=Left
  a : PMIOPort  Port=2  Side=Right
  b : PMIOPort  Port=3  Side=Right
  connections:
  b/RConn1 -- Phase Splitter2/RConn2
  abc/RConn1 -- Phase Splitter2/LConn1
  a/RConn1 -- Phase Splitter2/RConn1

== system MATE_IEEE123Node/NorthEast/sph40 ==
  Phase Splitter2 : ee_lib/Connectors & References/Phase Splitter
  abc : PMIOPort  Side=Left
  a : PMIOPort  Port=2  Side=Right
  connections:
  a/RConn1 -- Phase Splitter2/RConn1
  abc/RConn1 -- Phase Splitter2/LConn1

== system MATE_IEEE123Node/NorthEast/sph41 ==
  Phase Splitter2 : ee_lib/Connectors & References/Phase Splitter
  abc : PMIOPort  Side=Left
  a : PMIOPort  Port=2  Side=Right
  b : PMIOPort  Port=3  Side=Right
  connections:
  a/RConn1 -- Phase Splitter2/RConn1
  abc/RConn1 -- Phase Splitter2/LConn1
  Phase Splitter2/RConn2 -- b/RConn1

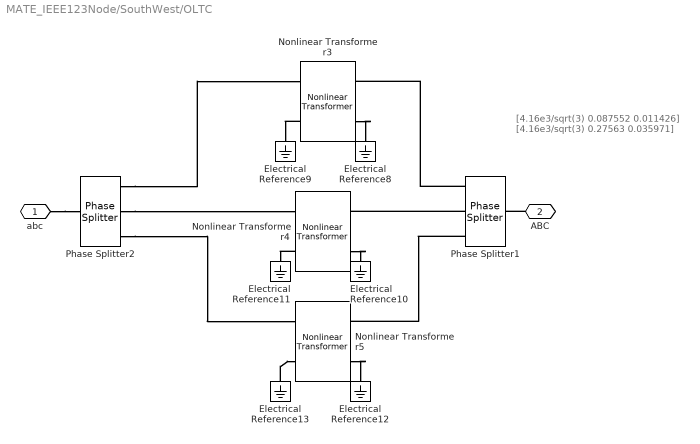
== system MATE_IEEE123Node/SouthWest/OLTC ==
  note: [4.16e3/sqrt(3) 0.087552 0.011426]
      | [4.16e3/sqrt(3) 0.27563 0.035971]
  Electrical Reference{8..13} (6 alike) : fl_lib/Electrical/Electrical Elements/Electrical Reference
  Nonlinear Transformer3 : ee_lib/Passive/Transformers/Nonlinear Transformer  Nw=1  Nw2=1  winding_param_option=2  Req=0.01 Ohm  Leq=0.0001 H  R_1=0.087552 Ohm  L_1=0.011426 H  R_2=0.27563 Ohm  L_2=0.035971 H  averaging_period=0 s  R_m=50000 Ohm  parameterization_option=1  H_data=[0, 200, 400, 600, 800, 1000] A/m  B_data=[0, .81, 1.25, 1.42, 1.48, 1.49] T  length_effective=0.2 m  area_effective=2e-4 m^2  L=1 H  L_sat=1e-2 H  current_data=[0, .4, .8, 1.2, 1.6, 2] A  magnetic_flux_data=[0, .161, .25, .284, .295, .299] .* 1e-3 Wb  magnetic_flux_sat=1.6e-04 Wb  dBdH0=0.005 T*m/A  B1=1.49 T  H1=1000 A/m  c=0.1  K=200 A/m  alpha=1e-4  interpolation_option=1  Leq_i0=0 A  L1_i0=0 A  L2_i0=0 A  x0_option=1  i_L0=0 A  phi0=0 Wb  B0=0 T  H0=0 A/m  Leq_g=1e-9 1/Ohm  L1_g=1e-9 1/Ohm  L2_g=1e-9 1/Ohm
      settings: InternalSimscapePortConfiguration="{\"Bottom\":[],\"Left\":[{\"id\":\"p1\",\"label\":\"1+\",\"type\":\"foundation.electrical.electrical\"},{\"id\":\"n1\",\"label\":\"1-\",\"type\":\"foundation.electrical.electrical\"}],\"Right\":[{\"id\":\"p2\",\"label\":\"2+\",\"type\":\"foundation.electrical.electrical\"},{\"id\":\"n2\",\"label\":\"2-\",\"type\":\"foundation.electrical.electrical\"}],\"Top\":[]}"
  Nonlinear Transformer4 : ee_lib/Passive/Transformers/Nonlinear Transformer  Nw=1  Nw2=1  winding_param_option=2  Req=0.01 Ohm  Leq=0.0001 H  R_1=0.087552 Ohm  L_1=0.011426 H  R_2=0.27563 Ohm  L_2=0.035971 H  averaging_period=0 s  R_m=50000 Ohm  parameterization_option=1  H_data=[0, 200, 400, 600, 800, 1000] A/m  B_data=[0, .81, 1.25, 1.42, 1.48, 1.49] T  length_effective=0.2 m  area_effective=2e-4 m^2  L=1 H  L_sat=1e-2 H  current_data=[0, .4, .8, 1.2, 1.6, 2] A  magnetic_flux_data=[0, .161, .25, .284, .295, .299] .* 1e-3 Wb  magnetic_flux_sat=1.6e-04 Wb  dBdH0=0.005 T*m/A  B1=1.49 T  H1=1000 A/m  c=0.1  K=200 A/m  alpha=1e-4  interpolation_option=1  Leq_i0=0 A  L1_i0=0 A  L2_i0=0 A  x0_option=1  i_L0=0 A  phi0=0 Wb  B0=0 T  H0=0 A/m  Leq_g=1e-9 1/Ohm  L1_g=1e-9 1/Ohm  L2_g=1e-9 1/Ohm
      settings: InternalSimscapePortConfiguration="{\"Bottom\":[],\"Left\":[{\"id\":\"p1\",\"label\":\"1+\",\"type\":\"foundation.electrical.electrical\"},{\"id\":\"n1\",\"label\":\"1-\",\"type\":\"foundation.electrical.electrical\"}],\"Right\":[{\"id\":\"p2\",\"label\":\"2+\",\"type\":\"foundation.electrical.electrical\"},{\"id\":\"n2\",\"label\":\"2-\",\"type\":\"foundation.electrical.electrical\"}],\"Top\":[]}"
  Nonlinear Transformer5 : ee_lib/Passive/Transformers/Nonlinear Transformer  Nw=1  Nw2=1  winding_param_option=2  Req=0.01 Ohm  Leq=0.0001 H  R_1=0.087552 Ohm  L_1=0.011426 H  R_2=0.27563 Ohm  L_2=0.035971 H  averaging_period=0 s  R_m=50000 Ohm  parameterization_option=1  H_data=[0, 200, 400, 600, 800, 1000] A/m  B_data=[0, .81, 1.25, 1.42, 1.48, 1.49] T  length_effective=0.2 m  area_effective=2e-4 m^2  L=1 H  L_sat=1e-2 H  current_data=[0, .4, .8, 1.2, 1.6, 2] A  magnetic_flux_data=[0, .161, .25, .284, .295, .299] .* 1e-3 Wb  magnetic_flux_sat=1.6e-04 Wb  dBdH0=0.005 T*m/A  B1=1.49 T  H1=1000 A/m  c=0.1  K=200 A/m  alpha=1e-4  interpolation_option=1  Leq_i0=0 A  L1_i0=0 A  L2_i0=0 A  x0_option=1  i_L0=0 A  phi0=0 Wb  B0=0 T  H0=0 A/m  Leq_g=1e-9 1/Ohm  L1_g=1e-9 1/Ohm  L2_g=1e-9 1/Ohm
      settings: InternalSimscapePortConfiguration="{\"Bottom\":[],\"Left\":[{\"id\":\"p1\",\"label\":\"1+\",\"type\":\"foundation.electrical.electrical\"},{\"id\":\"n1\",\"label\":\"1-\",\"type\":\"foundation.electrical.electrical\"}],\"Right\":[{\"id\":\"p2\",\"label\":\"2+\",\"type\":\"foundation.electrical.electrical\"},{\"id\":\"n2\",\"label\":\"2-\",\"type\":\"foundation.electrical.electrical\"}],\"Top\":[]}"
  Phase Splitter1 : ee_lib/Connectors & References/Phase Splitter
  Phase Splitter2 : ee_lib/Connectors & References/Phase Splitter
  abc : PMIOPort  Side=Left
  ABC : PMIOPort  Port=2  Side=Right
  connections:
  Nonlinear Transformer4/RConn2 -- Electrical Reference10/LConn1
  Nonlinear Transformer5/RConn2 -- Electrical Reference12/LConn1
  Electrical Reference13/LConn1 -- Nonlinear Transformer5/LConn2
  Nonlinear Transformer3/LConn2 -- Electrical Reference9/LConn1
  Nonlinear Transformer4/LConn2 -- Electrical Reference11/LConn1
  Nonlinear Transformer3/RConn2 -- Electrical Reference8/LConn1
  Phase Splitter2/RConn3 -- Nonlinear Transformer5/LConn1
  Phase Splitter2/RConn2 -- Nonlinear Transformer4/LConn1
  abc/RConn1 -- Phase Splitter2/LConn1
  Phase Splitter2/RConn1 -- Nonlinear Transformer3/LConn1
  ABC/RConn1 -- Phase Splitter1/LConn1
  Phase Splitter1/RConn1 -- Nonlinear Transformer3/RConn1
  Phase Splitter1/RConn2 -- Nonlinear Transformer4/RConn1
  Phase Splitter1/RConn3 -- Nonlinear Transformer5/RConn1

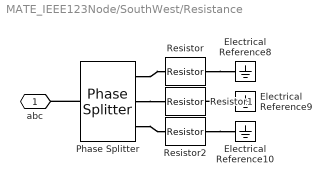
== system MATE_IEEE123Node/SouthWest/Resistance ==
  Electrical Reference10 : fl_lib/Electrical/Electrical Elements/Electrical Reference
  Electrical Reference8 : fl_lib/Electrical/Electrical Elements/Electrical Reference
  Electrical Reference9 : fl_lib/Electrical/Electrical Elements/Electrical Reference
  Phase Splitter : ee_lib/Connectors & References/Phase Splitter
  Resistor : ee_lib/Passive/Resistor  R=R(1) Ohm  enable_R_tol=ee.enum.toleranceApplication.none  R_tol=5  tol_distribution=ee.enum.toleranceDistribution.uniform  nSigma=4  enable_operating_limits=ee.enum.enable.no  operating_limit_action=ee.enum.passive.reportOpLim.warn  power_rating=1 W  max_working_voltage=100 V  noise_mode=ee.enum.sources.noise.Disabled  Tdevice=25 degC  sample_time=1e-3 s  repeatability=ee.enum.ic.repeatability.notRepeatable  user_seed=0  auto_seed=3499211588  fault_action=simscape.enum.assert.action.none  t_fault=1 s  power_derating_T1=70 degC  power_derating_T2=155 degC  operating_temperature_range_vec=[-50, 150] degC  alpha=3.93e-3 1/K  Tmeas=25 degC  thermal_mass=100 J/K  temperature_specify=off  temperature_priority=High  temperature=298.15 K  temperature_nominal_specify=off  temperature_nominal_value=1  temperature_nominal_unit=K
  Resistor1 : ee_lib/Passive/Resistor  R=R(2) Ohm  enable_R_tol=ee.enum.toleranceApplication.none  R_tol=5  tol_distribution=ee.enum.toleranceDistribution.uniform  nSigma=4  enable_operating_limits=ee.enum.enable.no  operating_limit_action=ee.enum.passive.reportOpLim.warn  power_rating=1 W  max_working_voltage=100 V  noise_mode=ee.enum.sources.noise.Disabled  Tdevice=25 degC  sample_time=1e-3 s  repeatability=ee.enum.ic.repeatability.notRepeatable  user_seed=0  auto_seed=3890346746  fault_action=simscape.enum.assert.action.none  t_fault=1 s  power_derating_T1=70 degC  power_derating_T2=155 degC  operating_temperature_range_vec=[-50, 150] degC  alpha=3.93e-3 1/K  Tmeas=25 degC  thermal_mass=100 J/K  temperature_specify=off  temperature_priority=High  temperature=298.15 K  temperature_nominal_specify=off  temperature_nominal_value=1  temperature_nominal_unit=K
  Resistor2 : ee_lib/Passive/Resistor  R=R(3) Ohm  enable_R_tol=ee.enum.toleranceApplication.none  R_tol=5  tol_distribution=ee.enum.toleranceDistribution.uniform  nSigma=4  enable_operating_limits=ee.enum.enable.no  operating_limit_action=ee.enum.passive.reportOpLim.warn  power_rating=1 W  max_working_voltage=100 V  noise_mode=ee.enum.sources.noise.Disabled  Tdevice=25 degC  sample_time=1e-3 s  repeatability=ee.enum.ic.repeatability.notRepeatable  user_seed=0  auto_seed=545404223  fault_action=simscape.enum.assert.action.none  t_fault=1 s  power_derating_T1=70 degC  power_derating_T2=155 degC  operating_temperature_range_vec=[-50, 150] degC  alpha=3.93e-3 1/K  Tmeas=25 degC  thermal_mass=100 J/K  temperature_specify=off  temperature_priority=High  temperature=298.15 K  temperature_nominal_specify=off  temperature_nominal_value=1  temperature_nominal_unit=K
  abc : PMIOPort  Side=Left
  connections:
  Phase Splitter/RConn2 -- Resistor1/LConn1
  Resistor/RConn1 -- Electrical Reference8/LConn1
  Phase Splitter/RConn3 -- Resistor2/LConn1
  Phase Splitter/LConn1 -- abc/RConn1
  Electrical Reference9/LConn1 -- Resistor1/RConn1
  Resistor2/RConn1 -- Electrical Reference10/LConn1
  Phase Splitter/RConn1 -- Resistor/LConn1

== system MATE_IEEE123Node/SouthWest/sph10 ==
  Phase Splitter2 : ee_lib/Connectors & References/Phase Splitter
  abc : PMIOPort  Side=Left
  c : PMIOPort  Port=2  Side=Right
  connections:
  Phase Splitter2/RConn3 -- c/RConn1
  abc/RConn1 -- Phase Splitter2/LConn1

== system MATE_IEEE123Node/SouthWest/sph11 ==
  Phase Splitter2 : ee_lib/Connectors & References/Phase Splitter
  abc : PMIOPort  Side=Left
  b : PMIOPort  Port=2  Side=Right
  connections:
  b/RConn1 -- Phase Splitter2/RConn2
  abc/RConn1 -- Phase Splitter2/LConn1

== system MATE_IEEE123Node/SouthWest/sph12 ==
  Phase Splitter2 : ee_lib/Connectors & References/Phase Splitter
  abc : PMIOPort  Side=Left
  b : PMIOPort  Port=2  Side=Right
  connections:
  abc/RConn1 -- Phase Splitter2/LConn1
  b/RConn1 -- Phase Splitter2/RConn2

== system MATE_IEEE123Node/SouthWest/sph13 ==
  Phase Splitter2 : ee_lib/Connectors & References/Phase Splitter
  abc : PMIOPort  Side=Left
  c : PMIOPort  Port=2  Side=Right
  connections:
  abc/RConn1 -- Phase Splitter2/LConn1
  Phase Splitter2/RConn3 -- c/RConn1

== system MATE_IEEE123Node/SouthWest/sph14 ==
  Phase Splitter2 : ee_lib/Connectors & References/Phase Splitter
  abc : PMIOPort  Side=Left
  a : PMIOPort  Port=2  Side=Right
  connections:
  abc/RConn1 -- Phase Splitter2/LConn1
  Phase Splitter2/RConn1 -- a/RConn1

== system MATE_IEEE123Node/SouthWest/sph15 ==
  Phase Splitter2 : ee_lib/Connectors & References/Phase Splitter
  abc : PMIOPort  Side=Left
  a : PMIOPort  Port=2  Side=Right
  connections:
  Phase Splitter2/RConn1 -- a/RConn1
  abc/RConn1 -- Phase Splitter2/LConn1

== system MATE_IEEE123Node/SouthWest/sph16 ==
  Phase Splitter2 : ee_lib/Connectors & References/Phase Splitter
  abc : PMIOPort  Side=Left
  b : PMIOPort  Port=2  Side=Right
  connections:
  abc/RConn1 -- Phase Splitter2/LConn1
  Phase Splitter2/RConn2 -- b/RConn1

== system MATE_IEEE123Node/SouthWest/sph17 ==
  Phase Splitter2 : ee_lib/Connectors & References/Phase Splitter
  abc : PMIOPort  Side=Left
  c : PMIOPort  Port=2  Side=Right
  connections:
  abc/RConn1 -- Phase Splitter2/LConn1
  Phase Splitter2/RConn3 -- c/RConn1

== system MATE_IEEE123Node/SouthWest/sph18 ==
  Phase Splitter2 : ee_lib/Connectors & References/Phase Splitter
  abc : PMIOPort  Side=Left
  c : PMIOPort  Port=2  Side=Right
  connections:
  Phase Splitter2/RConn3 -- c/RConn1
  abc/RConn1 -- Phase Splitter2/LConn1

== system MATE_IEEE123Node/SouthWest/sph19 ==
  Phase Splitter2 : ee_lib/Connectors & References/Phase Splitter
  abc : PMIOPort  Side=Left
  b : PMIOPort  Port=2  Side=Right
  connections:
  Phase Splitter2/RConn2 -- b/RConn1
  abc/RConn1 -- Phase Splitter2/LConn1

== system MATE_IEEE123Node/SouthWest/sph20 ==
  Phase Splitter2 : ee_lib/Connectors & References/Phase Splitter
  abc : PMIOPort  Side=Left
  a : PMIOPort  Port=2  Side=Right
  connections:
  abc/RConn1 -- Phase Splitter2/LConn1
  Phase Splitter2/RConn1 -- a/RConn1

== system MATE_IEEE123Node/SouthWest/sph45 ==
  Phase Splitter2 : ee_lib/Connectors & References/Phase Splitter
  abc : PMIOPort  Side=Left
  c : PMIOPort  Port=2  Side=Right
  connections:
  abc/RConn1 -- Phase Splitter2/LConn1
  Phase Splitter2/RConn3 -- c/RConn1

== system MATE_IEEE123Node/SouthWest/sph46 ==
  Phase Splitter2 : ee_lib/Connectors & References/Phase Splitter
  abc : PMIOPort  Side=Left
  a : PMIOPort  Port=2  Side=Right
  connections:
  abc/RConn1 -- Phase Splitter2/LConn1
  a/RConn1 -- Phase Splitter2/RConn1

== system MATE_IEEE123Node/SouthWest/sph47 ==
  Phase Splitter2 : ee_lib/Connectors & References/Phase Splitter
  abc : PMIOPort  Side=Left
  b : PMIOPort  Port=2  Side=Right
  connections:
  abc/RConn1 -- Phase Splitter2/LConn1
  Phase Splitter2/RConn2 -- b/RConn1

== system MATE_IEEE123Node/SouthWest/sph48 ==
  Phase Splitter2 : ee_lib/Connectors & References/Phase Splitter
  abc : PMIOPort  Side=Left
  c : PMIOPort  Port=2  Side=Right
  connections:
  abc/RConn1 -- Phase Splitter2/LConn1
  Phase Splitter2/RConn3 -- c/RConn1

== system MATE_IEEE123Node/SouthWest/sph49 ==
  Phase Splitter2 : ee_lib/Connectors & References/Phase Splitter
  abc : PMIOPort  Side=Left
  a : PMIOPort  Port=2  Side=Right
  connections:
  abc/RConn1 -- Phase Splitter2/LConn1
  Phase Splitter2/RConn1 -- a/RConn1

== system MATE_IEEE123Node/SouthWest/sph50 ==
  Phase Splitter2 : ee_lib/Connectors & References/Phase Splitter
  abc : PMIOPort  Side=Left
  c : PMIOPort  Port=2  Side=Right
  connections:
  abc/RConn1 -- Phase Splitter2/LConn1
  Phase Splitter2/RConn3 -- c/RConn1

== system MATE_IEEE123Node/SouthWest/sph52 ==
  Phase Splitter2 : ee_lib/Connectors & References/Phase Splitter
  abc : PMIOPort  Side=Left
  a : PMIOPort  Port=2  Side=Right
  connections:
  Phase Splitter2/RConn1 -- a/RConn1
  abc/RConn1 -- Phase Splitter2/LConn1

== system MATE_IEEE123Node/SouthWest/sph9 ==
  Phase Splitter2 : ee_lib/Connectors & References/Phase Splitter
  abc : PMIOPort  Side=Left
  a : PMIOPort  Port=2  Side=Right
  connections:
  abc/RConn1 -- Phase Splitter2/LConn1
  a/RConn1 -- Phase Splitter2/RConn1

== system MATE_IEEE123Node/MATEREF/MATE 3ph/SRC_CONI ==
  Conn1 : PMIOPort  Side=Left
  Conn2 : PMIOPort  Port=2  Side=Right
  connections:
  Conn1/RConn1 -- Conn2/RConn1

== system MATE_IEEE123Node/MATEREF/MATE 3ph/SRC_CONV ==
  Conn1 : PMIOPort  Side=Left
  Conn2 : PMIOPort  Port=2  Side=Right
  connections:
  Conn1/RConn1 -- Conn2/RConn1

== system MATE_IEEE123Node/MATEREF/MATE 3ph1/SRC_CONI ==
  Conn1 : PMIOPort  Side=Left
  Conn2 : PMIOPort  Port=2  Side=Right
  connections:
  Conn1/RConn1 -- Conn2/RConn1

== system MATE_IEEE123Node/MATEREF/MATE 3ph1/SRC_CONV ==
  Conn1 : PMIOPort  Side=Left
  Conn2 : PMIOPort  Port=2  Side=Right
  connections:
  Conn1/RConn1 -- Conn2/RConn1

== system MATE_IEEE123Node/MATEREF/MATE 3ph2/SRC_CONI ==
  Conn1 : PMIOPort  Side=Left
  Conn2 : PMIOPort  Port=2  Side=Right
  connections:
  Conn1/RConn1 -- Conn2/RConn1

== system MATE_IEEE123Node/MATEREF/MATE 3ph2/SRC_CONV ==
  Conn1 : PMIOPort  Side=Left
  Conn2 : PMIOPort  Port=2  Side=Right
  connections:
  Conn1/RConn1 -- Conn2/RConn1
